simulink model "model_moj_stara_verzija"  (R2021a)
settings: Solver=FixedStepAuto  StartTime=0.0  StopTime=450  FixedStep=0.01  RelTol=1e-3
undefined symbols (not defined in the file or in its folder): National_Instruments, PCIe
libraries: sldrtlib x4, slident x1
settings Model: Creator=lab  LastModifiedBy=zv210379d

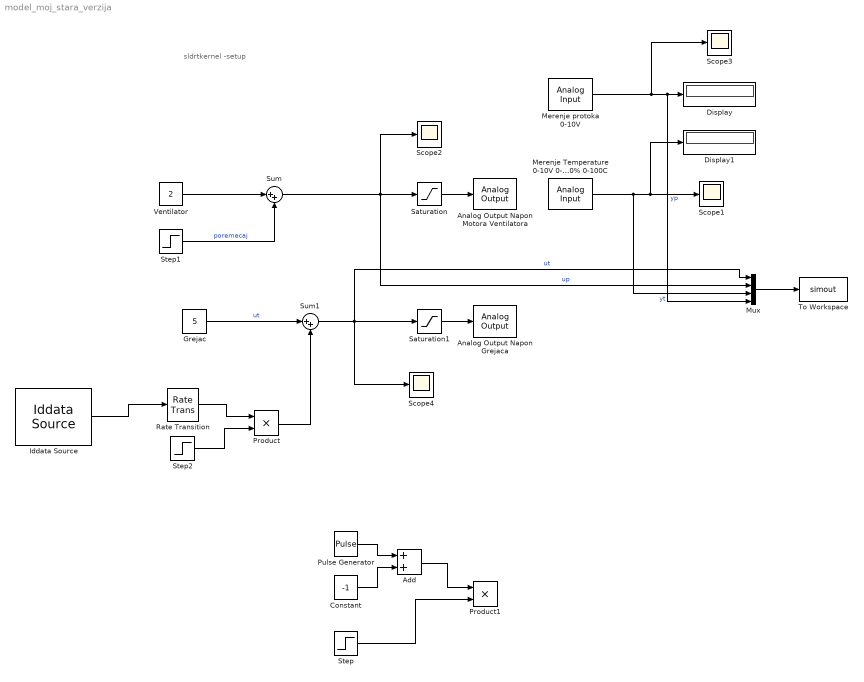
== system model_moj_stara_verzija ==
  note: sldrtkernel -setup
  Add : Sum
  Analog Output Napon Grejaca : sldrtlib/Analog Output  SampleTime=0.01  MaxMissedTicks=10000  ShowMissedTicks=off  YieldWhenWaiting=off  DrvName=National_Instruments/PCIe-6323  DrvAddress=4294967295  DrvOptions=[0 0 0 0 0 0 0]  Channels=2  RangeMode=1  VoltRange=1  InitialValue=0  FinalValue=0
      settings: AttributesFormatString=National Instruments\nPCIe-6323 [auto]
  Analog Output Napon Motora Ventilatora : sldrtlib/Analog Output  SampleTime=0.01  MaxMissedTicks=10000  ShowMissedTicks=off  YieldWhenWaiting=off  DrvName=National_Instruments/PCIe-6323  DrvAddress=4294967295  DrvOptions=[0 0 0 0 0 0 0]  Channels=1  RangeMode=1  VoltRange=1  InitialValue=[]  FinalValue=[]
      settings: AttributesFormatString=National Instruments\nPCIe-6323 [auto]
  Constant : Constant  Value=-1
  Display : Display
  Display1 : Display
  Grejac : Constant  Value=5
  Iddata Source : slident/Iddata Source  iddataobj=data
      settings: SourceProductBaseCode=ID
  Merenje Temperature 0-10V 0-100% 0-100C : sldrtlib/Analog Input  SampleTime=0.01  MaxMissedTicks=10000  ShowMissedTicks=off  YieldWhenWaiting=off  DrvName=National_Instruments/PCIe-6323  DrvAddress=4294967295  DrvOptions=[0 0 0 0 0 0 0]  Channels=3  RangeMode=1  VoltRange=1  DataType=1
      settings: AttributesFormatString=National Instruments\nPCIe-6323 [auto]
  Merenje protoka 0-10V : sldrtlib/Analog Input  SampleTime=0.01  MaxMissedTicks=10000  ShowMissedTicks=off  YieldWhenWaiting=on  DrvName=National_Instruments/PCIe-6323  DrvAddress=4294967295  DrvOptions=[0 0 0 0 0 0 0]  Channels=6  RangeMode=1  VoltRange=1  DataType=1
      settings: AttributesFormatString=National Instruments\nPCIe-6323 [auto]
  Mux : Mux
  Product : Product
  Product1 : Product
  Pulse Generator : DiscretePulseGenerator  PulseType=Time based  Amplitude=2  Period=20  PulseWidth=50
  Rate Transition : RateTransition
  Saturation : Saturate  UpperLimit=10  LowerLimit=0
  Saturation1 : Saturate  UpperLimit=10  LowerLimit=0
  Scope{1..4} (4 alike) : Scope
  Step : Step  Time=50  SampleTime=0
  Step1 : Step  Time=250  After=3  SampleTime=0
  Step2 : Step  Time=50  SampleTime=0
  Sum : Sum  Inputs=|++
  Sum1 : Sum  Inputs=|++
  To Workspace : ToWorkspace  VariableName=simout  SampleTime=0.01
  Ventilator : Constant  Value=2
  wires:
  Grejac/1 -> Sum1/1  "ut"
  Mux/1 -> To Workspace/1
  Saturation1/1 -> Analog Output Napon Grejaca/1
  Merenje protoka 0-10V/1 -> Display/1, Mux/4, Scope3/1  "yp"
  Saturation/1 -> Analog Output Napon Motora Ventilatora/1
  Ventilator/1 -> Sum/1
  Merenje Temperature 0-10V 0-100% 0-100C/1 -> Mux/3, Display1/1, Scope1/1  "yt"
  Step1/1 -> Sum/2  "poremecaj"
  Sum/1 -> Saturation/1, Mux/2, Scope2/1  "up"
  Sum1/1 -> Mux/1, Scope4/1, Saturation1/1  "ut"
  Iddata Source/1 -> Rate Transition/1
  Step2/1 -> Product/2
  Rate Transition/1 -> Product/1
  Pulse Generator/1 -> Add/1
  Constant/1 -> Add/2
  Add/1 -> Product1/1
  Step/1 -> Product1/2
  Product/1 -> Sum1/2
